simulink model "teslab1ex2"  (Simulink 7.2)
settings: Solver=ode45  StartTime=0.0  StopTime=10.0  RelTol=1e-3
undefined symbols (not defined in the file or in its folder): functieg
settings Model: Creator=Student  LastModifiedBy=Student

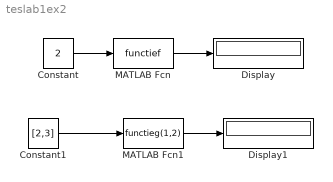
== system teslab1ex2 ==
  Constant : Constant  Value=2  OutDataType=sfix(16)  OutScaling=2^0
  Constant1 : Constant  Value=[2,3]  OutDataType=fixdt(1,16)  ConRadixGroup=Best Precision: Vector-wise
  Display : Display
  Display1 : Display
  MATLAB Fcn : MATLABFcn  MATLABFcn=functief
  MATLAB Fcn1 : MATLABFcn  MATLABFcn=functieg(1,2)
  wires:
  Constant/1 -> MATLAB Fcn/1
  MATLAB Fcn/1 -> Display/1
  MATLAB Fcn1/1 -> Display1/1
  Constant1/1 -> MATLAB Fcn1/1
